simulink model "SPGF_FSK_0000_R2022b"  (R2022b)
settings: Solver=ode4  StartTime=0.0  StopTime=1.4  FixedStep=50e-6/50  RelTol=1e-3  EnableMultiTasking=on
undefined symbols (not defined in the file): D11, Delta
libraries: spsSeriesRLCBranchLib x1646, spsGroundLib x360, spsStairGeneratorLib x147, spsIdealSwitchLib x145, spsCurrentMeasurementLib x145, spsUniversalBridgeLib x76, spsThreePhaseSeriesRLCLoadLib x57, simulink x45, spsBistableLib x36, spsSequenceAnalyzerLib x31, spsThreePhaseParallelRLCLoadLib x20, spsThreePhaseTransformerTwoWindingsLib x20
(part 40 of 40)

== system SPGF_FSK_0000_R2022b/K9/fault/Time Delay/SC_Time5/Triggered Subsystem1 ==
  Tr : Inport
  Time : Inport  Port=2
  Clock : Inport  Port=3
  Enable : EnablePort
  Add : Sum
  Memory3 : Memory  InheritSampleTime=on
  Memory4 : Memory  InheritSampleTime=on
  Relational Operator : RelationalOperator  Operator=>  OutDataTypeStr=boolean  InputSameDT=off
  Triggered Subsystem2 : Subsystem  TreatAsAtomicUnit=on
  Out : Outport  InitialOutput=0
  wires:
  Triggered Subsystem2/1(Out1) -> Add/1
  Add/1 -> Relational Operator/2
  Tr/1 -> Memory4/1
  Time/1 -> Add/2
  Relational Operator/1 -> Out/1
  Clock/1 -> Memory3/1, Triggered Subsystem2/1(In1)
  Memory3/1 -> Relational Operator/1
  Memory4/1 -> Triggered Subsystem2/Trigger

== system SPGF_FSK_0000_R2022b/spgf/Control/Arcing/ArcStrV/AddRamp ==
  SG : Inport
  Add1 : Sum
  Add2 : Sum  Inputs=+-
  Add3 : Sum  Inputs=+-
  Clock : Clock
  Memory1 : Memory
  Memory2 : Memory
  Product : Product
  Slopes : spsStairGeneratorLib/Stair Generator  t=SwitchTimesVoltageArc  e=SlopeInPattern  Ts=0
  Triggered Subsystem : Subsystem  TreatAsAtomicUnit=on
  O : Outport
  wires:
  Add1/1 -> O/1
  Memory2/1 -> Add2/2
  Product/1 -> Add1/2
  Slopes/1 -> Product/1
  Triggered Subsystem/1(O) -> Memory2/1
  Clock/1 -> Triggered Subsystem/1(I), Add2/1
  Memory1/1 -> Add3/2
  Add3/1 -> Triggered Subsystem/Trigger
  Add2/1 -> Product/2
  SG/1 -> Add3/1, Memory1/1, Add1/1

== system SPGF_FSK_0000_R2022b/spgf/Control/Arcing/ArcStrV/Pulse ==
  Add : Sum
  Constant : Constant  Value=VoltageArcBase
  Pulse Generator : DiscretePulseGenerator  PulseType=Time based  Amplitude=PulseAmpV  Period=PulsePeriodV  PulseWidth=PulseWidthV  PhaseDelay=PulsePhaseDelayV
  Scope : Scope
  O : Outport
  wires:
  Add/1 -> O/1
  Pulse Generator/1 -> Add/1, Scope/1
  Constant/1 -> Add/2

== system SPGF_FSK_0000_R2022b/spgf/Control/Arcing/Peters & Slepian/Filtering ==
  I : Inport
  Bistable1 : spsBistableLib/Bistable  Qpriority=Set  ic=0  Ts=0
      settings: LibrarySourceBlock=sps_lib/Control/Bistable
  Filter : spsSecondOrderFilterLib/Second-Order Filter  FilterType=Lowpass  Fo=FreqFilter  Zeta=0.707  Ts=0  Initialize=on  Vac_Init="[0,  0,  50]"  Vdc_Init=0  PlotResponse=off  FreqRange=[0, 500, 1]
      settings: LibrarySourceBlock=|
      | sps_lib/Control/Filters/Second-Order
      | Filter
  Memory1 : Memory
  On Delay : spsOnDelayLib/On Delay  DelayType=On delay  delay=FilterReturnTime  ic=0  Ts=0
  Terminator1 : Terminator
  Zero Crossing : Subsystem
  O : Outport
  wires:
  Bistable1/1 -> Memory1/1, O/1
  I/1 -> Filter/1
  On Delay/1 -> Bistable1/2
  Bistable1/2 -> Terminator1/1
  Memory1/1 -> On Delay/1
  Zero Crossing/1(O) -> Bistable1/1
  Filter/1 -> Zero Crossing/1(I)

== system SPGF_FSK_0000_R2022b/spgf/Control/Arcing/Peters & Slepian/Waiting ==
  Arc : Inport
  Add3 : Sum
  Clock : Clock
  Memory : Memory
  Relational Operator5 : RelationalOperator  OutDataTypeStr=boolean  InputSameDT=off
  Triggered Subsystem1 : Subsystem  TreatAsAtomicUnit=on
  WaitTime : Constant  Value=WaitTime
  O : Outport
  wires:
  Triggered Subsystem1/1(O) -> Add3/1
  Add3/1 -> Relational Operator5/2
  Memory/1 -> Triggered Subsystem1/Trigger
  Arc/1 -> Memory/1
  Clock/1 -> Triggered Subsystem1/1(I), Relational Operator5/1
  WaitTime/1 -> Add3/2
  Relational Operator5/1 -> O/1

== system SPGF_FSK_0000_R2022b/spgf/Control/Time Delay/SC_Time5/Triggered Subsystem1 ==
  Tr : Inport
  Time : Inport  Port=2
  Clock : Inport  Port=3
  Enable : EnablePort
  Add : Sum
  Memory3 : Memory  InheritSampleTime=on
  Memory4 : Memory  InheritSampleTime=on
  Relational Operator : RelationalOperator  Operator=>  OutDataTypeStr=boolean  InputSameDT=off
  Triggered Subsystem2 : Subsystem  TreatAsAtomicUnit=on
  Out : Outport  InitialOutput=0
  wires:
  Triggered Subsystem2/1(Out1) -> Add/1
  Add/1 -> Relational Operator/2
  Tr/1 -> Memory4/1
  Time/1 -> Add/2
  Relational Operator/1 -> Out/1
  Clock/1 -> Memory3/1, Triggered Subsystem2/1(In1)
  Memory3/1 -> Relational Operator/1
  Memory4/1 -> Triggered Subsystem2/Trigger

== system SPGF_FSK_0000_R2022b/K1/fault/Arcing/ArcStrV/AddRamp/Triggered Subsystem ==
  I : Inport
  Trigger : TriggerPort  TriggerType=either  VariantControl=(inherit)
  O : Outport
  wires:
  I/1 -> O/1

== system SPGF_FSK_0000_R2022b/K1/fault/Arcing/Peters & Slepian/Filtering/Zero Crossing ==
  I : Inport
  Compare To Zero : simulink/Logic and Bit Operations/Compare To Zero  relop=~=  OutDataTypeStr=boolean
  DTC_D1 : DataTypeConversion  OutDataTypeStr=double  SaturateOnIntegerOverflow=off  RndMeth=Floor
  Hit Crossing : HitCross
  Product1 : Product
  O : Outport
  wires:
  Product1/1 -> O/1
  DTC_D1/1 -> Product1/1
  Hit Crossing/1 -> Product1/2
  I/1 -> Compare To Zero/1, Hit Crossing/1
  Compare To Zero/1 -> DTC_D1/1

== system SPGF_FSK_0000_R2022b/K1/fault/Arcing/Peters & Slepian/Waiting/Triggered Subsystem1 ==
  I : Inport
  Trigger : TriggerPort  VariantControl=Variant
  O : Outport
  wires:
  I/1 -> O/1

== system SPGF_FSK_0000_R2022b/K1/fault/Time Delay/SC_Time5/Triggered Subsystem1/Triggered Subsystem2 ==
  In1 : Inport
  Trigger : TriggerPort  VariantControl=Variant
  Out1 : Outport  InitialOutput=0
  wires:
  In1/1 -> Out1/1

== system SPGF_FSK_0000_R2022b/K2/fault/Arcing/ArcStrV/AddRamp/Triggered Subsystem ==
  I : Inport
  Trigger : TriggerPort  TriggerType=either  VariantControl=(inherit)
  O : Outport
  wires:
  I/1 -> O/1

== system SPGF_FSK_0000_R2022b/K2/fault/Arcing/Peters & Slepian/Filtering/Zero Crossing ==
  I : Inport
  Compare To Zero : simulink/Logic and Bit Operations/Compare To Zero  relop=~=  OutDataTypeStr=boolean
  DTC_D1 : DataTypeConversion  OutDataTypeStr=double  SaturateOnIntegerOverflow=off  RndMeth=Floor
  Hit Crossing : HitCross
  Product1 : Product
  O : Outport
  wires:
  Product1/1 -> O/1
  DTC_D1/1 -> Product1/1
  Hit Crossing/1 -> Product1/2
  I/1 -> Compare To Zero/1, Hit Crossing/1
  Compare To Zero/1 -> DTC_D1/1

== system SPGF_FSK_0000_R2022b/K2/fault/Arcing/Peters & Slepian/Waiting/Triggered Subsystem1 ==
  I : Inport
  Trigger : TriggerPort  VariantControl=Variant
  O : Outport
  wires:
  I/1 -> O/1

== system SPGF_FSK_0000_R2022b/K2/fault/Time Delay/SC_Time5/Triggered Subsystem1/Triggered Subsystem2 ==
  In1 : Inport
  Trigger : TriggerPort  VariantControl=Variant
  Out1 : Outport  InitialOutput=0
  wires:
  In1/1 -> Out1/1

== system SPGF_FSK_0000_R2022b/K3/fault/Arcing/ArcStrV/AddRamp/Triggered Subsystem ==
  I : Inport
  Trigger : TriggerPort  TriggerType=either  VariantControl=(inherit)
  O : Outport
  wires:
  I/1 -> O/1

== system SPGF_FSK_0000_R2022b/K3/fault/Arcing/Peters & Slepian/Filtering/Zero Crossing ==
  I : Inport
  Compare To Zero : simulink/Logic and Bit Operations/Compare To Zero  relop=~=  OutDataTypeStr=boolean
  DTC_D1 : DataTypeConversion  OutDataTypeStr=double  SaturateOnIntegerOverflow=off  RndMeth=Floor
  Hit Crossing : HitCross
  Product1 : Product
  O : Outport
  wires:
  Product1/1 -> O/1
  DTC_D1/1 -> Product1/1
  Hit Crossing/1 -> Product1/2
  I/1 -> Compare To Zero/1, Hit Crossing/1
  Compare To Zero/1 -> DTC_D1/1

== system SPGF_FSK_0000_R2022b/K3/fault/Arcing/Peters & Slepian/Waiting/Triggered Subsystem1 ==
  I : Inport
  Trigger : TriggerPort  VariantControl=Variant
  O : Outport
  wires:
  I/1 -> O/1

== system SPGF_FSK_0000_R2022b/K3/fault/Time Delay/SC_Time5/Triggered Subsystem1/Triggered Subsystem2 ==
  In1 : Inport
  Trigger : TriggerPort  VariantControl=Variant
  Out1 : Outport  InitialOutput=0
  wires:
  In1/1 -> Out1/1

== system SPGF_FSK_0000_R2022b/K4/fault/Arcing/ArcStrV/AddRamp/Triggered Subsystem ==
  I : Inport
  Trigger : TriggerPort  TriggerType=either  VariantControl=(inherit)
  O : Outport
  wires:
  I/1 -> O/1

== system SPGF_FSK_0000_R2022b/K4/fault/Arcing/Peters & Slepian/Filtering/Zero Crossing ==
  I : Inport
  Compare To Zero : simulink/Logic and Bit Operations/Compare To Zero  relop=~=  OutDataTypeStr=boolean
  DTC_D1 : DataTypeConversion  OutDataTypeStr=double  SaturateOnIntegerOverflow=off  RndMeth=Floor
  Hit Crossing : HitCross
  Product1 : Product
  O : Outport
  wires:
  Product1/1 -> O/1
  DTC_D1/1 -> Product1/1
  Hit Crossing/1 -> Product1/2
  I/1 -> Compare To Zero/1, Hit Crossing/1
  Compare To Zero/1 -> DTC_D1/1

== system SPGF_FSK_0000_R2022b/K4/fault/Arcing/Peters & Slepian/Waiting/Triggered Subsystem1 ==
  I : Inport
  Trigger : TriggerPort  VariantControl=Variant
  O : Outport
  wires:
  I/1 -> O/1

== system SPGF_FSK_0000_R2022b/K4/fault/Time Delay/SC_Time5/Triggered Subsystem1/Triggered Subsystem2 ==
  In1 : Inport
  Trigger : TriggerPort  VariantControl=Variant
  Out1 : Outport  InitialOutput=0
  wires:
  In1/1 -> Out1/1

== system SPGF_FSK_0000_R2022b/K5/fault/Arcing/ArcStrV/AddRamp/Triggered Subsystem ==
  I : Inport
  Trigger : TriggerPort  TriggerType=either  VariantControl=(inherit)
  O : Outport
  wires:
  I/1 -> O/1

== system SPGF_FSK_0000_R2022b/K5/fault/Arcing/Peters & Slepian/Filtering/Zero Crossing ==
  I : Inport
  Compare To Zero : simulink/Logic and Bit Operations/Compare To Zero  relop=~=  OutDataTypeStr=boolean
  DTC_D1 : DataTypeConversion  OutDataTypeStr=double  SaturateOnIntegerOverflow=off  RndMeth=Floor
  Hit Crossing : HitCross
  Product1 : Product
  O : Outport
  wires:
  Product1/1 -> O/1
  DTC_D1/1 -> Product1/1
  Hit Crossing/1 -> Product1/2
  I/1 -> Compare To Zero/1, Hit Crossing/1
  Compare To Zero/1 -> DTC_D1/1

== system SPGF_FSK_0000_R2022b/K5/fault/Arcing/Peters & Slepian/Waiting/Triggered Subsystem1 ==
  I : Inport
  Trigger : TriggerPort  VariantControl=Variant
  O : Outport
  wires:
  I/1 -> O/1

== system SPGF_FSK_0000_R2022b/K5/fault/Time Delay/SC_Time5/Triggered Subsystem1/Triggered Subsystem2 ==
  In1 : Inport
  Trigger : TriggerPort  VariantControl=Variant
  Out1 : Outport  InitialOutput=0
  wires:
  In1/1 -> Out1/1

== system SPGF_FSK_0000_R2022b/K6/fault/Arcing/ArcStrV/AddRamp/Triggered Subsystem ==
  I : Inport
  Trigger : TriggerPort  TriggerType=either  VariantControl=(inherit)
  O : Outport
  wires:
  I/1 -> O/1

== system SPGF_FSK_0000_R2022b/K6/fault/Arcing/Peters & Slepian/Filtering/Zero Crossing ==
  I : Inport
  Compare To Zero : simulink/Logic and Bit Operations/Compare To Zero  relop=~=  OutDataTypeStr=boolean
  DTC_D1 : DataTypeConversion  OutDataTypeStr=double  SaturateOnIntegerOverflow=off  RndMeth=Floor
  Hit Crossing : HitCross
  Product1 : Product
  O : Outport
  wires:
  Product1/1 -> O/1
  DTC_D1/1 -> Product1/1
  Hit Crossing/1 -> Product1/2
  I/1 -> Compare To Zero/1, Hit Crossing/1
  Compare To Zero/1 -> DTC_D1/1

== system SPGF_FSK_0000_R2022b/K6/fault/Arcing/Peters & Slepian/Waiting/Triggered Subsystem1 ==
  I : Inport
  Trigger : TriggerPort  VariantControl=Variant
  O : Outport
  wires:
  I/1 -> O/1

== system SPGF_FSK_0000_R2022b/K6/fault/Time Delay/SC_Time5/Triggered Subsystem1/Triggered Subsystem2 ==
  In1 : Inport
  Trigger : TriggerPort  VariantControl=Variant
  Out1 : Outport  InitialOutput=0
  wires:
  In1/1 -> Out1/1

== system SPGF_FSK_0000_R2022b/K8/fault/Arcing/ArcStrV/AddRamp/Triggered Subsystem ==
  I : Inport
  Trigger : TriggerPort  TriggerType=either  VariantControl=(inherit)
  O : Outport
  wires:
  I/1 -> O/1

== system SPGF_FSK_0000_R2022b/K8/fault/Arcing/Peters & Slepian/Filtering/Zero Crossing ==
  I : Inport
  Compare To Zero : simulink/Logic and Bit Operations/Compare To Zero  relop=~=  OutDataTypeStr=boolean
  DTC_D1 : DataTypeConversion  OutDataTypeStr=double  SaturateOnIntegerOverflow=off  RndMeth=Floor
  Hit Crossing : HitCross
  Product1 : Product
  O : Outport
  wires:
  Product1/1 -> O/1
  DTC_D1/1 -> Product1/1
  Hit Crossing/1 -> Product1/2
  I/1 -> Compare To Zero/1, Hit Crossing/1
  Compare To Zero/1 -> DTC_D1/1

== system SPGF_FSK_0000_R2022b/K8/fault/Arcing/Peters & Slepian/Waiting/Triggered Subsystem1 ==
  I : Inport
  Trigger : TriggerPort  VariantControl=Variant
  O : Outport
  wires:
  I/1 -> O/1

== system SPGF_FSK_0000_R2022b/K8/fault/Time Delay/SC_Time5/Triggered Subsystem1/Triggered Subsystem2 ==
  In1 : Inport
  Trigger : TriggerPort  VariantControl=Variant
  Out1 : Outport  InitialOutput=0
  wires:
  In1/1 -> Out1/1

== system SPGF_FSK_0000_R2022b/K9/fault/Arcing/ArcStrV/AddRamp/Triggered Subsystem ==
  I : Inport
  Trigger : TriggerPort  TriggerType=either  VariantControl=(inherit)
  O : Outport
  wires:
  I/1 -> O/1

== system SPGF_FSK_0000_R2022b/K9/fault/Arcing/Peters & Slepian/Filtering/Zero Crossing ==
  I : Inport
  Compare To Zero : simulink/Logic and Bit Operations/Compare To Zero  relop=~=  OutDataTypeStr=boolean
  DTC_D1 : DataTypeConversion  OutDataTypeStr=double  SaturateOnIntegerOverflow=off  RndMeth=Floor
  Hit Crossing : HitCross
  Product1 : Product
  O : Outport
  wires:
  Product1/1 -> O/1
  DTC_D1/1 -> Product1/1
  Hit Crossing/1 -> Product1/2
  I/1 -> Compare To Zero/1, Hit Crossing/1
  Compare To Zero/1 -> DTC_D1/1

== system SPGF_FSK_0000_R2022b/K9/fault/Arcing/Peters & Slepian/Waiting/Triggered Subsystem1 ==
  I : Inport
  Trigger : TriggerPort  VariantControl=Variant
  O : Outport
  wires:
  I/1 -> O/1

== system SPGF_FSK_0000_R2022b/K9/fault/Time Delay/SC_Time5/Triggered Subsystem1/Triggered Subsystem2 ==
  In1 : Inport
  Trigger : TriggerPort  VariantControl=Variant
  Out1 : Outport  InitialOutput=0
  wires:
  In1/1 -> Out1/1

== system SPGF_FSK_0000_R2022b/spgf/Control/Arcing/ArcStrV/AddRamp/Triggered Subsystem ==
  I : Inport
  Trigger : TriggerPort  TriggerType=either  VariantControl=(inherit)
  O : Outport
  wires:
  I/1 -> O/1

== system SPGF_FSK_0000_R2022b/spgf/Control/Arcing/Peters & Slepian/Filtering/Zero Crossing ==
  I : Inport
  Compare To Zero : simulink/Logic and Bit Operations/Compare To Zero  relop=~=  OutDataTypeStr=boolean
  DTC_D1 : DataTypeConversion  OutDataTypeStr=double  SaturateOnIntegerOverflow=off  RndMeth=Floor
  Hit Crossing : HitCross
  Product1 : Product
  O : Outport
  wires:
  Product1/1 -> O/1
  DTC_D1/1 -> Product1/1
  Hit Crossing/1 -> Product1/2
  I/1 -> Compare To Zero/1, Hit Crossing/1
  Compare To Zero/1 -> DTC_D1/1

== system SPGF_FSK_0000_R2022b/spgf/Control/Arcing/Peters & Slepian/Waiting/Triggered Subsystem1 ==
  I : Inport
  Trigger : TriggerPort  VariantControl=Variant
  O : Outport
  wires:
  I/1 -> O/1

== system SPGF_FSK_0000_R2022b/spgf/Control/Time Delay/SC_Time5/Triggered Subsystem1/Triggered Subsystem2 ==
  In1 : Inport
  Trigger : TriggerPort  VariantControl=Variant
  Out1 : Outport  InitialOutput=0
  wires:
  In1/1 -> Out1/1
